simulink model "a_adaptiveSystemidentifikation"  (R2018b)
settings: Solver=ode45  StartTime=0.0  StopTime=30000.0  RelTol=1e-3  EnableMultiTasking=on
libraries: dspadpt3 x2, dspspect3 x2, simulink x2
settings Model: Creator=Wirnitzer  LastModifiedBy=Wirnitzer
settings DataIOCC: LimitDataPoints=on  SaveFormat=Array  SignalLoggingSaveFormat=ModelDataLogs
settings OptimizationCC: BooleanDataType=off  InitFltsAndDblsToZero=on  LifeSpan=inf
settings DebuggingCC: SaveWithParameterizedLinksMsg=none  UnderspecifiedInitializationDetection=Classic  MergeDetectMultiDrivingBlocksExec=none  SignalResolutionControl=TryResolveAllWithWarning  MultiTaskDSMMsg=warning  MultiTaskCondExecSysMsg=none  FcnCallInpInsideContextMsg=warning  SFUnexpectedBacktrackingDiag=warning  SFNoUnconditionalDefaultTransitionDiag=warning  SFExecutionAtInitializationDiag=none
settings HardwareCC: ProdBitPerPointer=32  ProdBitPerSizeT=32  ProdBitPerPtrDiffT=32  ProdLargestAtomicFloat=None  ProdIntDivRoundTo=Undefined  ProdEndianess=Unspecified  ProdWordSize=32  ProdHWDeviceType=32-bit Generic  TargetBitPerPointer=64  TargetBitPerSizeT=64  TargetBitPerPtrDiffT=64  TargetLongLongMode=on  TargetIntDivRoundTo=Zero  TargetEndianess=LittleEndian  TargetWordSize=64  TargetHWDeviceType=MATLAB Host  ProdEqTarget=off
settings ModelReferenceCC: PropagateSignalLabelsOutOfModel=off
settings SFSimCC: SimUseLocalCustomCode=off
settings RTWCC: RTWUseLocalCustomCode=off
settings CodeAppCC: StateflowObjectComments=on
settings GRTTargetCC: TargetFcnLib=ansi_tfl_tmw.mat  TargetLangStandard=C89/C90 (ANSI)  ModelReferenceCompliant=off  CombineOutputUpdateFcns=off  MatFileLogging=off  GRTInterface=on
settings ConfigComp: CovMetricSettings=dw  CovHtmlReporting=on  CovSaveCumulativeToWorkspaceVar=on  CovSaveSingleToWorkspaceVar=on  CovExternalEMLEnable=off

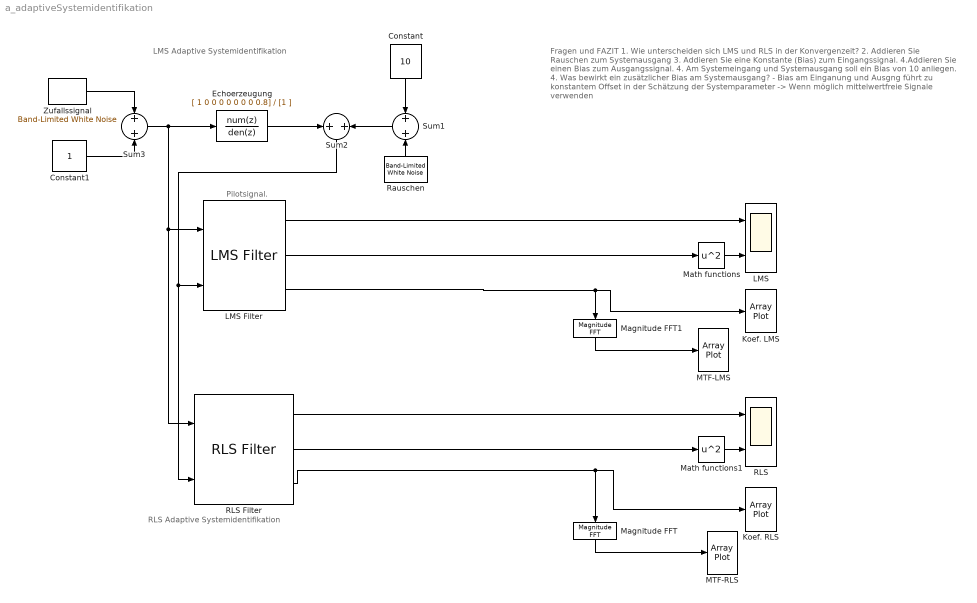
== system a_adaptiveSystemidentifikation ==
  note: Fragen und  FAZIT
      |
      | 1.  Wie unterscheiden sich LMS und RLS in der Konvergenzeit?
      |
      | 2. Addieren Sie Rauschen zum Systemausgang
      |
      |
      | 3. Addieren Sie eine Konstante (Bias) zum Eingangssignal.
      |
      | 4.Addieren Sie einen Bias zum Ausgangssignal.
      |
      |
      |
      | 4. Am Systemeingang und Systemausgang soll ein Bias von 10 anliegen.
      |
      | 4. Was bewirkt ein zusätzlicher Bias am Systemausgang?
      |
      | -  Bias am Einganung und Ausgng führt zu konstantem Offset in der Schätzung der Systemparameter  -> Wenn möglich mittelwertfreie Signale verwenden
  note: Pilotsignal.
  note: RLS Adaptive Systemidentifikation
  note: LMS Adaptive Systemidentifikation
  Constant : Constant  Value=10  SampleTime=1
  Constant1 : Constant  SampleTime=1
  Echoerzeugung : DiscreteFilter  Numerator=[ 1 0 0 0 0 0 0 0 0.8]  Denominator=[1 ]  SampleTime=1
  Koef. LMS : ArrayPlot
  Koef. RLS : ArrayPlot
  LMS : Scope  NumInputPorts=2
      settings: AttributesFormatString=test
  LMS Filter : dspadpt3/LMS Filter  Algo=Normalized LMS  L=50  stepflag=Dialog  mu=0.01  leakage=1  ic=0  Adapt=off  resetflag=None  weights=on  secondCoeffMode=User-defined  secondCoeffWordLength=2  secondCoeffFracLength=15  accum2Mode=User-defined  accum2FracLength=20  prodOutput2Mode=User-defined  prodOutput2FracLength=20  prodOutput3Mode=User-defined  prodOutput3FracLength=20  prodOutput4Mode=User-defined  prodOutput4FracLength=20  quotientMode=User-defined  quotientFracLength=20  roundingMode=Floor  overflowMode=off  addnparflag=off
      settings: SourceProductName=DSP System Toolbox  SourceProductBaseCode=DS
  MTF-LMS : ArrayPlot
  MTF-RLS : ArrayPlot
  Magnitude FFT : dspspect3/Magnitude FFT  mag_or_magsq=Magnitude  FFTImplementation=Auto  fftLenInherit=off  fftsize=256  WrapInput=on
      settings: SourceProductName=DSP System Toolbox  SourceProductBaseCode=DS
  Magnitude FFT1 : dspspect3/Magnitude FFT  mag_or_magsq=Magnitude  FFTImplementation=Auto  fftLenInherit=off  fftsize=256  WrapInput=on
      settings: SourceProductName=DSP System Toolbox  SourceProductBaseCode=DS
  Math functions : Math  Operator=square  SaturateOnIntegerOverflow=on
  Math functions1 : Math  Operator=square  SaturateOnIntegerOverflow=on
  RLS : Scope  NumInputPorts=2
  RLS Filter : dspadpt3/RLS Filter  L=50  lambdaflag=Dialog  lambda=0.99999  addnparflag=on  ic=0  delta=0.1  Adapt=off  resetflag=None  weights=on
      settings: SourceProductName=DSP System Toolbox  SourceProductBaseCode=DS
  Rauschen : simulink/Sources/Band-Limited White Noise  Cov=0.1  Ts=10  seed=[241]
  Sum1 : Sum  SaturateOnIntegerOverflow=on  InputSameDT=on  OutDataTypeStr=Inherit: Same as first input
  Sum2 : Sum  SaturateOnIntegerOverflow=on  InputSameDT=on  OutDataTypeStr=Inherit: Same as first input
  Sum3 : Sum  SaturateOnIntegerOverflow=on  InputSameDT=on  OutDataTypeStr=Inherit: Same as first input
  Zufallssignal : simulink/Sources/Band-Limited White Noise  Cov=1  Ts=1  seed=[23341]
  wires:
  Math functions/1 -> LMS/2
  LMS Filter/1 -> LMS/1
  LMS Filter/2 -> Math functions/1
  LMS Filter/3 -> Koef. LMS/1, Magnitude FFT1/1
  Math functions1/1 -> RLS/2
  RLS Filter/1 -> RLS/1
  RLS Filter/2 -> Math functions1/1
  RLS Filter/3 -> Koef. RLS/1, Magnitude FFT/1
  Magnitude FFT/1 -> MTF-RLS/1
  Magnitude FFT1/1 -> MTF-LMS/1
  Rauschen/1 -> Sum1/2
  Zufallssignal/1 -> Sum3/1
  Constant1/1 -> Sum3/2
  Sum3/1 -> RLS Filter/1, LMS Filter/1, Echoerzeugung/1
  Echoerzeugung/1 -> Sum2/1
  Sum2/1 -> RLS Filter/2, LMS Filter/2
  Constant/1 -> Sum1/1
  Sum1/1 -> Sum2/2
